simulink model "esoTest"  (R2016b)
settings: Solver=VariableStepAuto  StartTime=0.0  StopTime=30  RelTol=1e-3
settings Model: Creator=lenovo  LastModifiedBy=lenovo

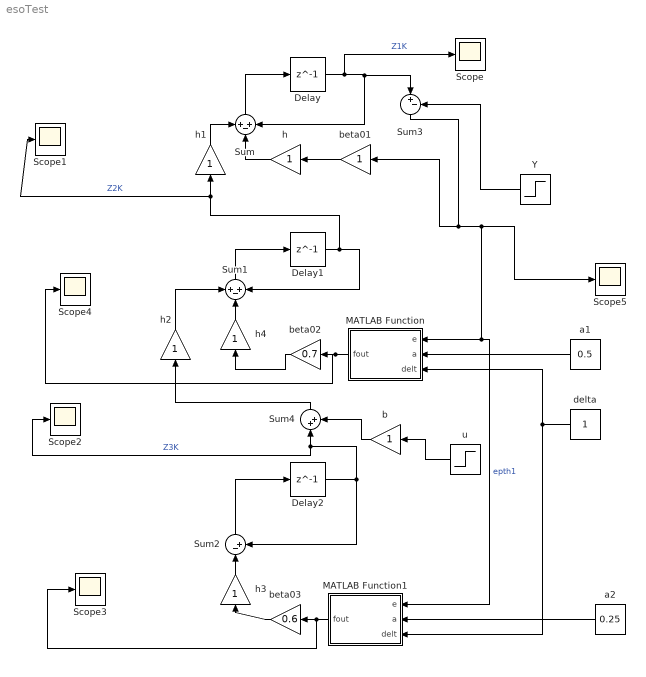
== system esoTest ==
  Delay : Delay  DelayLength=1
  Delay1 : Delay  DelayLength=1
  Delay2 : Delay  DelayLength=1
  MATLAB Function : MATLAB Function  TreatAsAtomicUnit=on
  MATLAB Function1 : MATLAB Function  TreatAsAtomicUnit=on
  Scope{,1..5} (6 alike) : Scope
  Sum : Sum  Inputs=+-+
  Sum1 : Sum  Inputs=+-+
  Sum2 : Sum  Inputs=|-+
  Sum3 : Sum  Inputs=|+-
  Sum4 : Sum  Inputs=|++
  Y : Step  Time=3  After=10  SampleTime=0
  a1 : Constant  Value=0.5
  a2 : Constant  Value=0.25
  b : Gain
  beta01 : Gain
  beta02 : Gain  Gain=0.7
  beta03 : Gain  Gain=0.6
  delta : Constant
  h{,1..4} (5 alike) : Gain
  u : Step  Time=5  After=10  SampleTime=0
  wires:
  Sum/1 -> Delay/1
  Delay/1 -> Scope/1, Sum3/1, Sum/3  "Z1K"
  Delay1/1 -> Scope1/1, h1/1, Sum1/3  "Z2K"
  Sum1/1 -> Delay1/1
  Delay2/1 -> Sum2/2, Scope2/1, Sum4/1  "Z3K"
  Sum2/1 -> Delay2/1
  Sum3/1 -> beta01/1, MATLAB Function1/1(e), MATLAB Function/1(e), Scope5/1  "epth1"
  h/1 -> Sum/2
  h1/1 -> Sum/1
  h2/1 -> Sum1/1
  Sum4/1 -> h2/1
  b/1 -> Sum4/2
  MATLAB Function1/1(fout) -> Scope3/1, beta03/1
  h3/1 -> Sum2/1
  beta03/1 -> h3/1
  a1/1 -> MATLAB Function/2(a)
  a2/1 -> MATLAB Function1/2(a)
  delta/1 -> MATLAB Function1/3(delt), MATLAB Function/3(delt)
  MATLAB Function/1(fout) -> Scope4/1, beta02/1
  beta01/1 -> h/1
  u/1 -> b/1
  Y/1 -> Sum3/2
  h4/1 -> Sum1/2
  beta02/1 -> h4/1

== matlab function esoTest/MATLAB Function1 ==
  data: e input; fout output; a input; delt input
function fout= falfcn(e,a,delt)
if abs(e)<=delt
    temp=1-a;
    fal=e/(delt^temp);
    
else
    
    fal=(abs(e))^a*sign(e);
end
fout=fal;

end

== matlab function esoTest/MATLAB Function ==
  data: e input; fout output; a input; delt input
function fout= falfcn(e,a,delt)
if abs(e)>delt
    fal=(abs(e))^a*sign(e);
else
    fal=delt^(1-a);
    fal=e/fal;
end
fout=fal;

end
